simulink model "active_state_sim"  (R2021b)
settings: Solver=VariableStepAuto  StartTime=0.0  StopTime=3  RelTol=1e-3
values from neighbouring files (symbols this model uses):
  a = K/B    (= 2.47037099211)    [active_state.m]
  b = K    (= 1471.6)    [active_state.m]
  c = (K*C)/B    (= 2765.82736277)    [active_state.m]
  d = K/B    (= 2.47037099211)    [active_state.m]
undefined symbols (not defined in the file or in its folder): sigbuilder_block
settings Model: Creator=eraym  LastModifiedBy=eraym

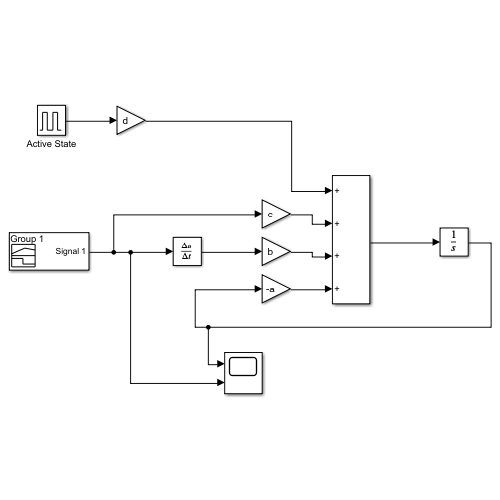
[thumbnail: Simulink's stored preview of the top-level diagram]
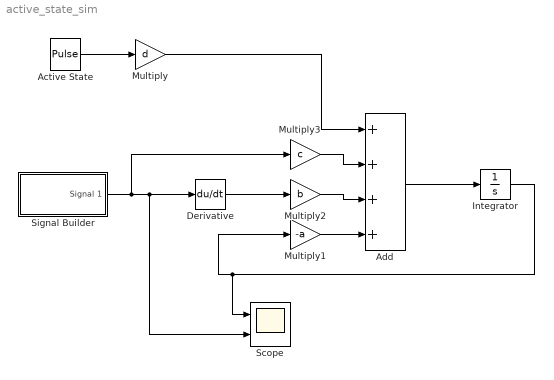
== system active_state_sim ==
  Active State : DiscretePulseGenerator  PulseType=Time based  Period=10  PulseWidth=5
  Add : Sum  Inputs=++++
  Derivative : Derivative
  Integrator : Integrator
  Multiply : Gain  Gain=d
  Multiply1 : Gain  Gain=-a
  Multiply2 : Gain  Gain=b
  Multiply3 : Gain  Gain=c
  Scope : Scope  NumInputPorts=2
  Signal Builder : Subsystem  Tag=STV Subsys  LoadFcn=sigbuilder_block('load');  StartFcn=sigbuilder_block('start');  StopFcn=sigbuilder_block('stop');  ClipboardFcn=sigbuilder_block('clipboard');  mask(Sigbuilder block){tuvar=[0:10]}
      mask help: Simulink:masks:SigbuilderBlock_MD
      mask init:
      | if ~strcmp(get_param(bdroot(gcbh),'SimulationStatus'),'stopped') tuvar = sigbuilder_block('maskInit'); end
      settings: CopyFcn=sigbuilder_block('copy');  DeleteFcn=sigbuilder_block('delete');  ModelCloseFcn=sigbuilder_block('modelClose');  PreSaveFcn=sigbuilder_block('preSave');  PauseFcn=sigbuilder_block('pause');  ContinueFcn=sigbuilder_block('continue');  NameChangeFcn=sigbuilder_block('namechange');  OpenFcn=sigbuilder_block('open',[633 207 550.5 399.75 ]);  CloseFcn=sigbuilder_block('close');
      mask Display: plot(0, 0, 100, 100,[2, 2, 32, 32, 2], [68, 8, 8, 68, 68],[32, 2], [38, 38], [32, 19, 2],[53, 60, 44], [32, 17, 17, 2],[16, 16, 31, 31]);txt = getActiveGroup(gcbh);text(2, 100, txt,'verticalAlignment', 'top');
  wires:
  Add/1 -> Integrator/1
  Active State/1 -> Multiply/1
  Multiply/1 -> Add/1
  Multiply1/1 -> Add/4
  Multiply2/1 -> Add/3
  Multiply3/1 -> Add/2
  Derivative/1 -> Multiply2/1
  Signal Builder/1(Signal 1) -> Multiply3/1, Scope/2, Derivative/1
  Integrator/1 -> Scope/1, Multiply1/1

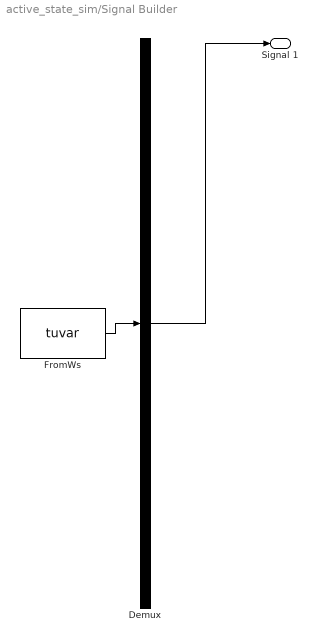
== system active_state_sim/Signal Builder ==
  Demux : Demux  Tag=STV Demux  Outputs=1
      settings: DisplayOption=none
  FromWs : FromWorkspace  Tag=STV FromWs  VariableName=tuvar
      SigBuilderData=|
      | common.afterFinalStr = 'Extrapolate'
      | common.sampleTime = 0
      | dataSet.timeRange = [0 10]
      | dataSet.name = 'Group 1'
      | sbobj.Groups.Name = 'Group 1'
      | sbobj.Groups.Signals.Name = 'Signal 1'
      | sbobj.Groups.Signals.XData = [0 1 1 2.02 2.02 10]
      | sbobj.Groups.Signals.YData = [0 0 1 1 0 0]
  Signal 1 : Outport  Tag=STV Outport
  wires:
  Demux/1 -> Signal 1/1
  FromWs/1 -> Demux/1
